simulink model "automata_learning"  (R2022a)
settings: Solver=FixedStepAuto  StartTime=0.0  StopTime=10.0  FixedStep=0.05  RelTol=1e-3
settings Model: Creator=diego  LastModifiedBy=diego

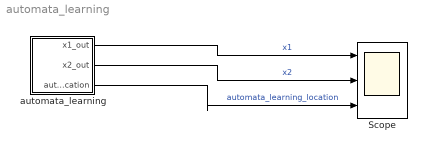
== system automata_learning ==
  Scope : Scope  NumInputPorts=3
  automata_learning : Stateflow chart  TreatAsAtomicUnit=on
  wires:
  automata_learning/1(x1_out) -> Scope/1  "x1"
  automata_learning/2(x2_out) -> Scope/2  "x2"
  automata_learning/3(automata_learning_location) -> Scope/3  "automata_learning_location"

== stateflow chart automata_learning/automata_learning ==
  settings: updateMethod=CONTINUOUS
  state loc1
    du:
    x1_dot = 54674876419.0 * x1 * x2 / 2305843009213694000.0 - 53162286057.0 * x2 / 1152921504606846980.0 - 4986999627.0 * x1 / 281474976710656.0 + 8639540389.0 * x1 ^ 2.0 / 2251799813685248.0 + 617091417.0 * x2 ^ 2.0 / 36893488147419103000.0 + 1.0000176972466388;
    x2_dot = 4503581376076071.0 * x1 / 4503599627370496.0 - 13133867609.0 * x2 / 2305843009213694000.0 + 11376815311.0 * x1 * x2 / 2305843009213694000.0 + 92691138733.0 * x1 ^ 2.0 / 72057594037927936.0 + 4617080777.0 * x2 ^ 2.0 / 295147905179352830000.0 + 0.0000018410548132397064;
    x1_out=x1;
    x2_out=x2;
    automata_learning_location =1;
  state loc2
    du:
    x1_dot = 145211639.0 * x1 / 4398046511104.0 - 7036799687709.0 * x2 / 140737488355328.0 - 317966099.0 * x1 * x2 / 2251799813685248.0 - 602871029.0 * x1 ^ 2.0 / 140737488355328.0 - 43990649.0 * x2 ^ 2.0 / 288230376151711740.0 - 0.0000634889212278722;
    x2_dot = 180223901.0 * x1 * x2 / 4503599627370496.0 - 176002231.0 * x2 / 1125899906842624.0 - 674003615.0 * x1 / 70368744177664.0 + 166242189.0 * x1 ^ 2.0 / 140737488355328.0 - 56764227.0 * x2 ^ 2.0 / 576460752303423490.0 + 1.0000193672808564;
    x1_out=x1;
    x2_out=x2;
    automata_learning_location =2;
  loc1 -> loc2 : [0.0000005511 * x2 - 0.2482 * x1 + 1.0 < 0.0]
  (default) -> loc1 : {x1 = 0.0;
      | x2 = 0.0;}
  loc2 -> loc1 : [43.09132960916031 * x1 + 0.021145646542095164 * x2 + 1.0 < 0.0 && -75.02048562094569 * x1 - 0.1991395009226835 * x2 + 1.0 > 0.0]
  data: x1_out output; x1 local; x2_out output; x2 local; automata_learning_location output
  data x1 settings: updateMethod=SF_CONTINUOUS_TIME_DATA
  data x2 settings: updateMethod=SF_CONTINUOUS_TIME_DATA
